simulink subsystem "MultibodySuspensionRearSSC"  (R2024b)
settings: Solver=VariableStepAuto  StartTime=0.0  StopTime=10.0  RelTol=1e-3
undefined symbols (not defined in the file): EnvGrvty, LAc, LAf, LAr, PlntVehDstCGFrntAxl, PlntVehDstCGRearAxl, PlntVehMass, PlntVehMultiBody, PlntVehMultiBodyGeom, RearRef, StrRodRL, UAc, UAf, UAr, Wheels, WhlAng, X, Y, Z
libraries: sm_lib x225, fl_lib x48, nesl_utility x32, sdl_lib x4
(part 1 of 9)
settings Model: ModifiedByFormat=The MathWorks, Inc.  Creator=The MathWorks, Inc.  LastModifiedBy=The MathWorks, Inc.
settings OptimizationCC: ReuseModelBlockBuffer=off
settings DebuggingCC: SubsystemReferenceDiagnosticForUnitTest=warning
settings RTWCC: GPUComputeCapability=3.5

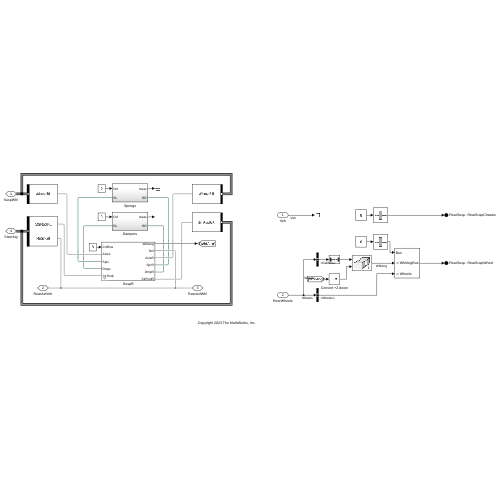
[thumbnail: Simulink's stored preview of the top-level diagram]
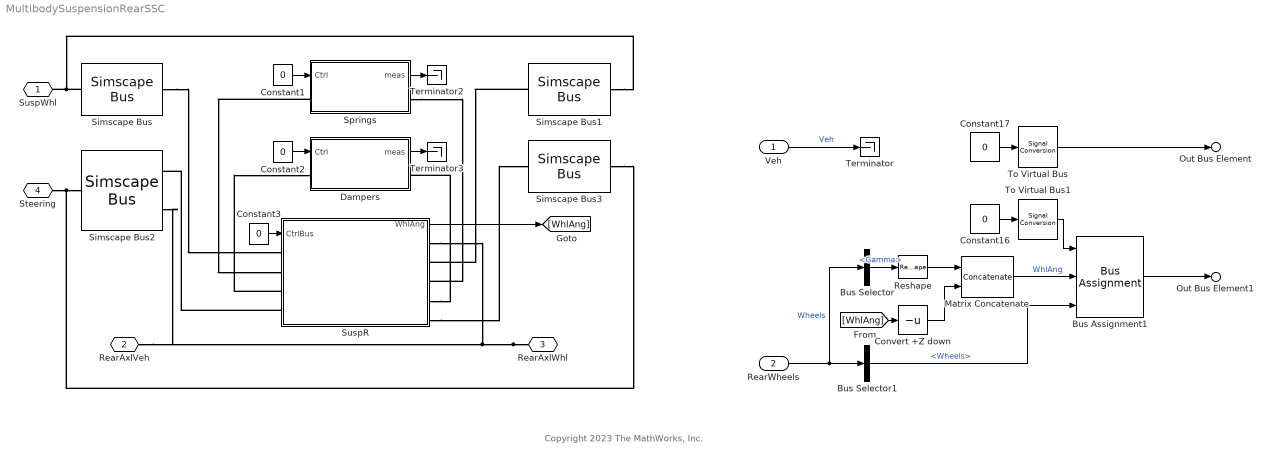
== system MultibodySuspensionRearSSC ==
  note: Copyright 2023 The MathWorks, Inc.
  Veh : Inport
  RearWheels : Inport  Port=2
  Bus Assignment1 : BusAssignment  AssignedSignals=WhlAng,Wheels
  Bus Selector : BusSelector  OutputSignals=Wheels.Gamma
  Bus Selector1 : BusSelector  OutputSignals=Wheels
  Constant1 : Constant  Value=0  SampleTime=-1
  Constant16 : Constant  Value=0  OutDataTypeStr=Bus: RearSuspWheelBUS  SampleTime=Inf
  Constant17 : Constant  Value=0  OutDataTypeStr=Bus: RearSuspChassisBUS  SampleTime=Inf
  Constant2 : Constant  Value=0  SampleTime=-1
  Constant3 : Constant  Value=0  SampleTime=-1
  Convert +Z down : UnaryMinus
  Dampers : Subsystem
  Matrix Concatenate : Concatenate  Mode=Multidimensional array
  Reshape : Reshape  OutputDimensionality=Row vector (2-D)
  Simscape Bus : SimscapeBus  HierarchyStrings=WheelRL
  Simscape Bus1 : SimscapeBus  HierarchyStrings=WheelRR
  Simscape Bus2 : SimscapeBus  HierarchyStrings=StrRodRL;RearRef
  Simscape Bus3 : SimscapeBus  HierarchyStrings=StrRodRR
  Springs : Subsystem
  SuspR : Subsystem  mask(Suspension and Steering){Susp=PlntVehMultiBody.Chassis.SuspR, Init=[0 0 0], InitTriggerDropdown=1}
      mask prompts: Susp "Suspension Parameters"; Init "Initial Values"; InitTriggerDropdown "Initialization Trigger Dropdown"
      mask help: Suspension and steering system for front or rear axle.
      mask init:
      | % curblk = gcb;
      | % Trigger Mask Initialization for 
      | % variant subsystems below this level
      | % sm_car_4post_lib_maskInitTrigger(curblk)
      settings: LibrarySourceBlock=sm_car_4post_lib/Suspension and Steering
      mask TypeOptions InitTriggerDropdown: 0 | 1
  Terminator : Terminator
  Terminator2 : Terminator
  Terminator3 : Terminator
  To Virtual Bus : SignalConversion  ConversionOutput=Virtual bus  OverrideOpt=off
  To Virtual Bus1 : SignalConversion  ConversionOutput=Virtual bus  OverrideOpt=off
  SuspWhl : PMIOPort  Side=Right
  RearAxlVeh : PMIOPort  Port=2  Side=Left
  RearAxlWhl : PMIOPort  Port=3  Side=Right
  Steering : PMIOPort  Port=4  Side=Left
  Out Bus Element : Outport  PortName=RearSusp  Element=RearSuspChassis
  Out Bus Element1 : Outport  PortName=RearSusp  Element=RearSuspWheel
  wires:
  Springs/1(meas) -> Terminator2/1
  Dampers/1(meas) -> Terminator3/1
  Constant1/1 -> Springs/1(Ctrl)
  Constant2/1 -> Dampers/1(Ctrl)
  Constant3/1 -> SuspR/1(CtrlBus)
  Bus Selector/1 -> Reshape/1  "<Gamma>"
  Reshape/1 -> Matrix Concatenate/1
  Convert +Z down/1 -> Matrix Concatenate/2
  SuspR/1(WhlAng) -> [WhlAng]
  [WhlAng] -> Convert +Z down/1
  Constant16/1 -> To Virtual Bus1/1
  To Virtual Bus/1 -> Out Bus Element/1
  Matrix Concatenate/1 -> Bus Assignment1/2  "WhlAng"
  Bus Assignment1/1 -> Out Bus Element1/1
  RearWheels/1 -> Bus Selector1/1, Bus Selector/1  "Wheels"
  Constant17/1 -> To Virtual Bus/1
  To Virtual Bus1/1 -> Bus Assignment1/1
  Bus Selector1/1 -> Bus Assignment1/3  "<Wheels>"
  Veh/1 -> Terminator/1  "Veh"
  connections:
  Steering/RConn1 -- Simscape Bus2/RConn1 -- Simscape Bus3/RConn1
  RearAxlWhl/RConn1 -- RearAxlVeh/RConn1 -- Simscape Bus2/LConn2 -- SuspR/RConn1
  Simscape Bus/RConn1 -- SuspWhl/RConn1 -- Simscape Bus1/RConn1
  SuspR/LConn4 -- Simscape Bus2/LConn1
  SuspR/RConn5 -- Simscape Bus3/LConn1
  Springs/LConn1 -- SuspR/LConn2
  Springs/RConn1 -- SuspR/RConn3
  SuspR/RConn4 -- Dampers/RConn1
  SuspR/LConn3 -- Dampers/LConn1
  Simscape Bus/LConn1 -- SuspR/LConn1
  Simscape Bus1/LConn1 -- SuspR/RConn2

== system MultibodySuspensionRearSSC/Dampers ==
  Ctrl : Inport
  Independent : Subsystem  VariantControl=Independent
  Terminator : Terminator
  RL : PMIOPort  Side=Left
  RR : PMIOPort  Port=2  Side=Right
  meas : Outport  VectorParamsAs1DForOutWhenUnconnected=off
  wires:
  Ctrl/1 -> Terminator/1
  Independent/1(meas) -> meas/1
  connections:
  Independent/RConn1 -- RR/RConn1
  Independent/LConn1 -- RL/RConn1

== system MultibodySuspensionRearSSC/Springs ==
  Ctrl : Inport
  Independent : Subsystem  VariantControl=Independent
  Terminator : Terminator
  RL : PMIOPort  Side=Left
  RR : PMIOPort  Port=2  Side=Right
  meas : Outport  VectorParamsAs1DForOutWhenUnconnected=off
  wires:
  Ctrl/1 -> Terminator/1
  Independent/1(meas) -> meas/1
  connections:
  Independent/RConn1 -- RR/RConn1
  Independent/LConn1 -- RL/RConn1

== system MultibodySuspensionRearSSC/SuspR ==
  CtrlBus : Inport
  Linkage : Subsystem  VariantControl=Linkage
  Terminator : Terminator
  AxleL : PMIOPort  Side=Left
  Ref : PMIOPort  Port=2  Side=Right
  AxleR : PMIOPort  Port=3  Side=Right
  SprL : PMIOPort  Port=4  Side=Left
  SprR : PMIOPort  Port=5  Side=Right
  DmpL : PMIOPort  Port=6  Side=Left
  DmpR : PMIOPort  Port=7  Side=Right
  StrRodL : PMIOPort  Port=8  Side=Left
  StrRodR : PMIOPort  Port=9  Side=Right
  WhlAng : Outport
  wires:
  Linkage/1(WhlAng) -> WhlAng/1
  CtrlBus/1 -> Terminator/1
  connections:
  Linkage/RConn5 -- StrRodR/RConn1
  StrRodL/RConn1 -- Linkage/LConn4
  Linkage/LConn1 -- AxleL/RConn1
  Linkage/RConn1 -- Ref/RConn1
  Linkage/RConn3 -- SprR/RConn1
  Linkage/RConn4 -- DmpR/RConn1
  Linkage/LConn2 -- SprL/RConn1
  Linkage/RConn2 -- AxleR/RConn1
  Linkage/LConn3 -- DmpL/RConn1

== system MultibodySuspensionRearSSC/Dampers/Independent ==
  Constant2 : Constant  Value=0  SampleTime=-1
  Constant3 : Constant  Value=0  SampleTime=-1
  Damper RL : Subsystem  mask(Damper){Damper=PlntVehMultiBody.Chassis.Damper.Rear}
      mask prompts: Damper "Damper Parameters"
      settings: LibrarySourceBlock=sm_car_4post_lib/Damper
  Damper RR : Subsystem  mask(Damper){Damper=PlntVehMultiBody.Chassis.Damper.Rear}
      mask prompts: Damper "Damper Parameters"
      settings: LibrarySourceBlock=sm_car_4post_lib/Damper
  MTRef RL : fl_lib/Mechanical/Translational Elements/Mechanical Translational Reference
  MTRef RR : fl_lib/Mechanical/Translational Elements/Mechanical Translational Reference
  RL : PMIOPort  Side=Left
  RR : PMIOPort  Port=2  Side=Right
  Out Bus Element2 : Outport  VectorParamsAs1DForOutWhenUnconnected=off  PortName=meas  Element=RL
  Out Bus Element3 : Outport  VectorParamsAs1DForOutWhenUnconnected=off  PortName=meas  Element=RR
  wires:
  Constant3/1 -> Damper RR/1(Ctrl)
  Constant2/1 -> Damper RL/1(Ctrl)
  Damper RR/1(meas) -> Out Bus Element3/1
  Damper RL/1(meas) -> Out Bus Element2/1
  connections:
  Damper RL/RConn1 -- MTRef RL/LConn1
  Damper RL/LConn1 -- RL/RConn1
  Damper RR/RConn1 -- MTRef RR/LConn1
  Damper RR/LConn1 -- RR/RConn1

== system MultibodySuspensionRearSSC/Springs/Independent ==
  Constant2 : Constant  Value=0  SampleTime=-1
  Constant3 : Constant  Value=0  SampleTime=-1
  MTRef RL : fl_lib/Mechanical/Translational Elements/Mechanical Translational Reference
  MTRef RR : fl_lib/Mechanical/Translational Elements/Mechanical Translational Reference
  Spring RL : Subsystem  mask(Spring){Spring=PlntVehMultiBody.Chassis.Spring.Rear}
      mask prompts: Spring "Spring Parameters"
      settings: LibrarySourceBlock=sm_car_4post_lib/Spring
  Spring RR : Subsystem  mask(Spring){Spring=PlntVehMultiBody.Chassis.Spring.Rear}
      mask prompts: Spring "Spring Parameters"
      settings: LibrarySourceBlock=sm_car_4post_lib/Spring
  RL : PMIOPort  Side=Left
  RR : PMIOPort  Port=2  Side=Right
  Out Bus Element2 : Outport  VectorParamsAs1DForOutWhenUnconnected=off  PortName=meas  Element=RL
  Out Bus Element3 : Outport  VectorParamsAs1DForOutWhenUnconnected=off  PortName=meas  Element=RR
  wires:
  Constant3/1 -> Spring RR/1(Ctrl)
  Constant2/1 -> Spring RL/1(Ctrl)
  Spring RR/1(meas) -> Out Bus Element3/1
  Spring RL/1(meas) -> Out Bus Element2/1
  connections:
  Spring RL/RConn1 -- MTRef RL/LConn1
  Spring RL/LConn1 -- RL/RConn1
  Spring RR/RConn1 -- MTRef RR/LConn1
  Spring RR/LConn1 -- RR/RConn1

== system MultibodySuspensionRearSSC/SuspR/Linkage ==
  Anti Roll Bar : Subsystem  Variant=on  VariantControlMode=label  LabelModeActiveChoice=Simple  mask{AntiRollBar=Susp.AntiRollBar, VariantLabel=Susp.AntiRollBar.class.Value, InitTriggerDropdown=1}
      mask prompts: AntiRollBar "Anti-Roll Bar"; VariantLabel "Variant Label"; InitTriggerDropdown "Initialization Trigger Dropdown"
      settings: AttributesFormatString=%<LabelModeActiveChoice>
      mask TypeOptions InitTriggerDropdown: 0 | 1
  Linkage L : Subsystem  Variant=on  VariantControlMode=label  VariantControl=Variant1  LabelModeActiveChoice=DoubleWishbone  mask(Suspension){popup_leftRight=Left, Linkage=Susp.Linkage, Init=[0 0 0], VariantLabel=Susp.Linkage.class.Value, InitTriggerDropdown=1}
      mask prompts: popup_leftRight "Left/Right"; Linkage "Linkage Parameters"; Init "Initial Values"; VariantLabel "Variant Label"; InitTriggerDropdown "Initialization Trigger Dropdown"
      mask help: Suspension with multiple variants. Variants are configured by parameter Variant Label. Parameter values are contained within Linkage Parameters.
      mask init:
      | % curblk = gcb;
      | 
      | % Set variant for this block 
      | % set_param(curblk,'LabelModeActiveChoice',VariantLabel);
      | 
      | % Trigger Mask Initialization for 
      | % variant subsystems below this level
      | % sm_car_4post_lib_maskInitTrigger(curblk)
      | 
      | % Set Left/Right fields
      | 
      | % sm_car_4post_lib_setLeftRight(curblk,'variant');
      settings: AttributesFormatString=%<ActiveVariant>  LibrarySourceBlock=sm_car_4post_lib/Suspension and Steering/Linkage/Linkage L
      mask TypeOptions popup_leftRight: Left | Right
      mask TypeOptions InitTriggerDropdown: 0 | 1
  Linkage R : Subsystem  Variant=on  VariantControlMode=label  VariantControl=Variant1  LabelModeActiveChoice=DoubleWishbone  mask(Suspension){popup_leftRight=Right, Linkage=Susp.Linkage, Init=[0 0 0], VariantLabel=Susp.Linkage.class.Value, InitTriggerDropdown=1}
      mask prompts: popup_leftRight "Left/Right"; Linkage "Linkage Parameters"; Init "Initial Values"; VariantLabel "Variant Label"; InitTriggerDropdown "Initialization Trigger Dropdown"
      mask help: Suspension with multiple variants. Variants are configured by parameter Variant Label. Parameter values are contained within Linkage Parameters.
      mask init:
      | % curblk = gcb;
      | 
      | % % Set variant for this block 
      | % set_param(curblk,'LabelModeActiveChoice',VariantLabel);
      | 
      | % Trigger Mask Initialization for 
      | % variant subsystems below this level
      | % sm_car_4post_lib_maskInitTrigger(curblk)
      | 
      | % Set Left/Right fields
      | 
      | % sm_car_4post_lib_setLeftRight(curblk,'variant');
      settings: AttributesFormatString=%<ActiveVariant>  LibrarySourceBlock=sm_car_4post_lib/Suspension and Steering/Linkage/Linkage R
      mask TypeOptions popup_leftRight: Left | Right
      mask TypeOptions InitTriggerDropdown: 0 | 1
  Matrix Concatenate : Concatenate  Mode=Multidimensional array  ConcatenateDimension=2
  AxleL : PMIOPort  Side=Left
  Ref : PMIOPort  Port=2  Side=Right
  AxleR : PMIOPort  Port=3  Side=Right
  SprL : PMIOPort  Port=4  Side=Left
  SprR : PMIOPort  Port=5  Side=Right
  DmpL : PMIOPort  Port=6  Side=Left
  DmpR : PMIOPort  Port=7  Side=Right
  StrRodL : PMIOPort  Port=8  Side=Left
  StrRodR : PMIOPort  Port=9  Side=Right
  WhlAng : Outport
  wires:
  Matrix Concatenate/1 -> WhlAng/1
  Linkage R/1(WhlAng) -> Matrix Concatenate/2
  Linkage L/1(WhlAng) -> Matrix Concatenate/1
  connections:
  Anti Roll Bar/LConn3 -- Linkage R/LConn4
  Anti Roll Bar/LConn1 -- Linkage L/LConn4
  Linkage R/LConn2 -- SprR/RConn1
  Linkage R/LConn3 -- DmpR/RConn1
  Linkage R/RConn1 -- StrRodR/RConn1
  Ref/RConn1 -- Anti Roll Bar/LConn2 -- Linkage L/RConn2 -- Linkage R/RConn2
  Linkage L/LConn1 -- AxleL/RConn1
  Linkage R/LConn1 -- AxleR/RConn1
  Linkage L/LConn2 -- SprL/RConn1
  Linkage L/LConn3 -- DmpL/RConn1
  Linkage L/RConn1 -- StrRodL/RConn1

== system MultibodySuspensionRearSSC/Dampers/Independent/Damper RL ==
  Ctrl : Inport
  Damper : Subsystem  Variant=on  VariantControlMode=label  VariantControl=Linear  LabelModeActiveChoice=Linear
  R : PMIOPort  Side=Left
  C : PMIOPort  Port=2  Side=Right
  meas : Outport  VectorParamsAs1DForOutWhenUnconnected=off
  wires:
  Damper/1(meas) -> meas/1
  Ctrl/1 -> Damper/1(Ctrl)
  connections:
  Damper/LConn1 -- R/RConn1
  Damper/RConn1 -- C/RConn1

== system MultibodySuspensionRearSSC/Dampers/Independent/Damper RR ==
  Ctrl : Inport
  Damper : Subsystem  Variant=on  VariantControlMode=label  VariantControl=Linear  LabelModeActiveChoice=Linear
  R : PMIOPort  Side=Left
  C : PMIOPort  Port=2  Side=Right
  meas : Outport  VectorParamsAs1DForOutWhenUnconnected=off
  wires:
  Damper/1(meas) -> meas/1
  Ctrl/1 -> Damper/1(Ctrl)
  connections:
  Damper/LConn1 -- R/RConn1
  Damper/RConn1 -- C/RConn1

== system MultibodySuspensionRearSSC/Springs/Independent/Spring RL ==
  Ctrl : Inport
  Spring : Subsystem  Variant=on  VariantControlMode=label  VariantControl=Linear  LabelModeActiveChoice=Linear
  R : PMIOPort  Side=Left
  C : PMIOPort  Port=2  Side=Right
  meas : Outport  VectorParamsAs1DForOutWhenUnconnected=off
  wires:
  Ctrl/1 -> Spring/1(Ctrl)
  Spring/1(meas) -> meas/1
  connections:
  Spring/RConn1 -- C/RConn1
  Spring/LConn1 -- R/RConn1

== system MultibodySuspensionRearSSC/Springs/Independent/Spring RR ==
  Ctrl : Inport
  Spring : Subsystem  Variant=on  VariantControlMode=label  VariantControl=Linear  LabelModeActiveChoice=Linear
  R : PMIOPort  Side=Left
  C : PMIOPort  Port=2  Side=Right
  meas : Outport  VectorParamsAs1DForOutWhenUnconnected=off
  wires:
  Ctrl/1 -> Spring/1(Ctrl)
  Spring/1(meas) -> meas/1
  connections:
  Spring/RConn1 -- C/RConn1
  Spring/LConn1 -- R/RConn1

== system MultibodySuspensionRearSSC/SuspR/Linkage/Anti Roll Bar ==
  " None" : Subsystem  VariantControl=None  mask(Anti-Roll Bar Placeholder){}
      mask help: Empty subsystem, used as a variant that omits an anti-roll bar.
  Simple : Subsystem  VariantControl=Simple  mask(Anti-Roll Bar, Simple){k=AntiRollBar.k.Value}
      mask prompts: k "Stiffness"
      mask help: Models an anti-roll bar by applying un-opposed forces to suspension arms. Conceptual use only.
  LAoL : PMIOPort  Side=Left
  Ref : PMIOPort  Port=2  Side=Left
  LAoR : PMIOPort  Port=3  Side=Left

== system MultibodySuspensionRearSSC/SuspR/Linkage/Linkage L ==
  DoubleWishbone : Subsystem  VariantControl=DoubleWishbone  mask(Double-Wishbone Suspension){popup_leftRight=Left, hp_in_f_ua=Linkage.UpperWishbone.sInboardF.Value, hp_in_r_ua=Linkage.UpperWishbone.sInboardR.Value, hp_out_ua=Linkage.UpperWishbone.sOutboard.Value, hp_in_f_la=Linkage.LowerWishbone.sInboardF.Value, hp_in_r_la=Linkage.LowerWishbone.sInboardR.Value, hp_out_la=Linkage.LowerWishbone.sOutboard.Value, hp_upr_cg=Linkage.Upright.sCG.Value, hp_upr_wc=Linkage.Upright.sWheelCentre.Value, hp_in_rod=Linkage.TrackRod.sInboard.Value, hp_upr_rod=Linkage.TrackRod.sOutboard.Value, hp_spr_top=Linkage.Shock.sTop.Value, hp_spr_bot=Linkage.Shock.sBottom.Value, clr_hp=PlntVehMultiBodyGeom.hp.clr, opc_hp=PlntVehMultiBodyGeom.hp.opc, size_hp=0.025, ua_mass=Linkage.UpperWishbone.m.Value, clr_ua=PlntVehMultiBodyGeom.yellow, opc_ua=PlntVehMultiBodyGeom.part.opc, radius_ua=0.02, la_mass=Linkage.LowerWishbone.m.Value, clr_la=PlntVehMultiBodyGeom.yellow, opc_la=PlntVehMultiBodyGeom.part.opc, radius_la=0.02, shock_pist_mass=Linkage.Shock.mPiston.Value, shock_cyl_mass=Linkage.Shock.mCylinder.Value, up_lim_bumpstop=Linkage.Endstop.xMax.Value, low_lim_bumpstop=Linkage.Endstop.xMin.Value, clr_conn_shock=PlntVehMultiBodyGeom.hp.clr, opc_conn_shock=PlntVehMultiBodyGeom.hp.opc, size_conn_shock=0.025, clr_shock_cyl=PlntVehMultiBodyGeom.blue, opc_shock_cyl=1.0, radius_shock_cyl=0.05, clr_shock_piston=PlntVehMultiBodyGeom.gray, opc_shock_piston=1.0, clr_shock_bumpstop=PlntVehMultiBodyGeom.yellowpale, opc_shock_bumpstop=1.0, deadvol_len_shock_cyl=PlntVehMultiBodyGeom.shock.dead_length, piston_len_shock=PlntVehMultiBodyGeom.shock.piston, cyl_cap_len_shock=PlntVehMultiBodyGeom.shock.cap, bumpstop_len_shock=PlntVehMultiBodyGeom.shock.bumpstop_len, upr_mass=Linkage.Upright.m.Value, atoe=Linkage.Upright.aToe.Value, acamber=Linkage.Upright.aCamber.Value, clr_conn_upr=PlntVehMultiBodyGeom.hp.clr, opc_conn_upr=PlntVehMultiBodyGeom.hp.opc, size_conn_upr=PlntVehMultiBodyGeom.hp.rad, clr_upr=PlntVehMultiBodyGeom.green, opc_upr=PlntVehMultiBodyGeom.part.opc, radius_upr=0.02, clr_stub_axle=PlntVehMultiBodyGeom.black, opc_stub_axle=PlntVehMultiBodyGeom.part.opc, radius_stub_axle=0.02, rod_mass=Linkage.TrackRod.m.Value, clr_conn_rod=PlntVehMultiBodyGeom.hp.clr, opc_conn_rod=PlntVehMultiBodyGeom.hp.opc, size_conn_rod=PlntVehMultiBodyGeom.hp.rad, clr_rod=PlntVehMultiBodyGeom.purple, opc_rod=PlntVehMultiBodyGeom.part.opc, radius_rod=0.02, whl_init_spd_lr=[0 0 0], whlind=1}
      mask prompts: popup_leftRight "Left/Right"; hp_in_f_ua "Upper Arm Front [xyz] (m)"; hp_in_r_ua "Upper Arm Rear [xyz] (m)"; hp_out_ua "Upper Arm Outboard [xyz] (m)"; hp_in_f_la "Lower Arm Front [xyz] (m)"; hp_in_r_la "Lower Arm Rear [xyz] (m)"; hp_out_la "Lower Arm Outboard [xyz] (m)"; hp_upr_cg "Upright CG [xyz] (m)"; hp_upr_wc "Wheel Center [xyz] (m)"; hp_in_rod "Track Rod Inboard [xyz] (m)"; hp_upr_rod "Track Rod Outboard [xyz] (m)"; hp_spr_top "Spring Top [xyz] (m)"; hp_spr_bot "Spring Bottom [xyz] (m)"; ua_mass "Mass (kg)"; clr_ua "Color [RGB]"; opc_ua "Opacity (0-1)"; radius_ua "Radius (m)"; la_mass "Mass (kg)"; clr_la "Color [RGB]"; opc_la "Opacity (0-1)"; radius_la "Radius (m)"; shock_pist_mass "Piston Mass (kg)"; shock_cyl_mass "Cylinder Mass (kg)"; up_lim_bumpstop "Upper Limit (m)"; low_lim_bumpstop "Lower Limit (m)"; deadvol_len_shock_cyl "Dead Volume Height (m)"; piston_len_shock "Piston Length (m)"; cyl_cap_len_shock "Cylinder Cap Length (m)"; bumpstop_len_shock "Bumpstop Length (m)"; upr_mass "Mass (kg)"; atoe "Toe Angle (deg)"; acamber "Camber Angle (deg)"; rod_mass "Mass (kg)"; whl_init_spd_lr "Initial Wheel Speed (rad/s)"; whlind "Wheel Index"
      mask help: This models a double-wishbone suspension for steered and non-steered configurations. The non-steered configuration maintains its orientation via the track rods that connect to fixed points on the subframe.
      mask init:
      | % sm_car_4post_lib_setLeftRight(gcb,'none');
      | 
      | if(popup_leftRight == 1)
      |     rhs_susp = 1;
      |     whlind = 1;
      | elseif(popup_leftRight == 2)
      |     rhs_susp = -1;
      |     whlind = 2;
      | end
      mask TypeOptions popup_leftRight: Left | Right
      mask TypeOptions hp_in_f_ua: Upper Arm/hp_in_f | Hardpoints/hp_in_f_ua
      mask TypeOptions hp_in_r_ua: Upper Arm/hp_in_r | Hardpoints/hp_in_r_ua
      mask TypeOptions hp_out_ua: Upper Arm/hp_out | Upright/hp_ua_out
      mask TypeOptions hp_in_f_la: Lower Arm/hp_in_f | Hardpoints/hp_in_f_la
      mask TypeOptions hp_in_r_la: Lower Arm/hp_in_r | Hardpoints/hp_in_r_la
      mask TypeOptions hp_out_la: Lower Arm/hp_out | Upright/hp_la_out
      mask TypeOptions hp_upr_cg: Upright/hp_upr_cg
      mask TypeOptions hp_upr_wc: Upright/hp_upr_wc
      mask TypeOptions hp_in_rod: Track Rod/hp_in
      mask TypeOptions hp_upr_rod: Track Rod/hp_out | Upright/hp_upr_rod
      mask TypeOptions hp_spr_top: Hardpoints/hp_spr_top | Shock/hp_spr_top
      mask TypeOptions hp_spr_bot: Lower Arm/hp_spr | Shock/hp_spr_bot
      mask TypeOptions clr_hp: Hardpoints/clr_hp
      mask TypeOptions opc_hp: Hardpoints/opc_hp
      mask TypeOptions size_hp: Hardpoints/size_hp
      mask TypeOptions ua_mass: Upper Arm/ua_mass
      mask TypeOptions clr_ua: Upper Arm/clr_ua
      mask TypeOptions opc_ua: Upper Arm/opc_ua
      mask TypeOptions radius_ua: Upper Arm/radius_ua
      mask TypeOptions la_mass: Lower Arm/la_mass
      mask TypeOptions clr_la: Lower Arm/clr_la
      mask TypeOptions opc_la: Lower Arm/opc_la
      mask TypeOptions radius_la: Lower Arm/radius_la
      mask TypeOptions shock_pist_mass: Shock/shock_pist_mass
      mask TypeOptions shock_cyl_mass: Shock/shock_cyl_mass
      mask TypeOptions up_lim_bumpstop: Shock/up_lim_bumpstop
      mask TypeOptions low_lim_bumpstop: Shock/low_lim_bumpstop
      mask TypeOptions clr_conn_shock: Shock/clr_conn_shock
      mask TypeOptions opc_conn_shock: Shock/opc_conn_shock
      mask TypeOptions size_conn_shock: Shock/size_conn_shock
      mask TypeOptions clr_shock_cyl: Shock/clr_shock_cyl
      mask TypeOptions opc_shock_cyl: Shock/opc_shock_cyl
      mask TypeOptions radius_shock_cyl: Shock/radius_shock_cyl
      mask TypeOptions clr_shock_piston: Shock/clr_shock_piston
      mask TypeOptions opc_shock_piston: Shock/opc_shock_piston
      mask TypeOptions clr_shock_bumpstop: Shock/clr_shock_bumpstop
      mask TypeOptions opc_shock_bumpstop: Shock/opc_shock_bumpstop
      mask TypeOptions deadvol_len_shock_cyl: Shock/deadvol_len_shock_cyl
      mask TypeOptions piston_len_shock: Shock/piston_len_shock
      mask TypeOptions cyl_cap_len_shock: Shock/cyl_cap_len_shock
      mask TypeOptions bumpstop_len_shock: Shock/bumpstop_len_shock
      mask TypeOptions upr_mass: Upright/upr_mass
      mask TypeOptions atoe: Upright/atoe
      mask TypeOptions acamber: Upright/acamber
      mask TypeOptions clr_conn_upr: Upright/clr_conn_upr
      mask TypeOptions opc_conn_upr: Upright/opc_conn_upr
      mask TypeOptions size_conn_upr: Upright/size_conn_upr
      mask TypeOptions clr_upr: Upright/clr_upr
      mask TypeOptions opc_upr: Upright/opc_upr
      mask TypeOptions radius_upr: Upright/radius_upr
      mask TypeOptions clr_stub_axle: Upright/clr_stub_axle
      mask TypeOptions opc_stub_axle: Upright/opc_stub_axle
      mask TypeOptions radius_stub_axle: Upright/radius_stub_axle
      mask TypeOptions rod_mass: Track Rod/rod_mass
      mask TypeOptions clr_conn_rod: Track Rod/clr_conn_rod
      mask TypeOptions opc_conn_rod: Track Rod/opc_conn_rod
      mask TypeOptions size_conn_rod: Track Rod/size_conn_rod
      mask TypeOptions clr_rod: Track Rod/clr_rod
      mask TypeOptions opc_rod: Track Rod/opc_rod
      mask TypeOptions radius_rod: Track Rod/radius_rod
      mask DialogControl cont_hp Prompt: Hardpoints
      mask DialogControl cont_vis_hp Prompt: Visualization
      mask DialogControl text_clr_hp Prompt: Color [RGB]
      mask DialogControl text_opc_hp Prompt: Opac. (0-1)
      mask DialogControl text_size_hp Prompt: Size (m)
      mask DialogControl text_hp Prompt: Hardpoints
      mask DialogControl cont_ua Prompt: UA
      mask DialogControl cont_vis_ua Prompt: Visualization
      mask DialogControl cont_la Prompt: LA
      mask DialogControl cont_vis_la Prompt: Visualization
      mask DialogControl cont_shock Prompt: Shock
      mask DialogControl cont_parts Prompt: Parts
      mask DialogControl cont_bumpstop Prompt: Bumpstop
      mask DialogControl cont_vis_shock Prompt: Visualization
      mask DialogControl text_clr_shock Prompt: Color  [RGB]
      mask DialogControl text_opc_shock Prompt: Opac. (0-1)
      mask DialogControl text_size_shock Prompt: Size (m)
      mask DialogControl text_conn_shock Prompt: Connections
      mask DialogControl text_shock_shock Prompt: Cylinder
      mask DialogControl text_shock_piston Prompt: Piston
      mask DialogControl text_piston_radius Prompt: <cylinder radius>
      mask DialogControl text_shock_bumpstop Prompt: Bumpstop
      mask DialogControl text_bumpstop_radius Prompt: <cylinder radius>
      mask DialogControl cont_upright Prompt: Upright
      mask DialogControl grp_upright Prompt: Upright
      mask DialogControl cont_vis_upr Prompt: Visualization
      mask DialogControl text_clr_upr Prompt: Color [RGB]
      mask DialogControl text_opc_upr Prompt: Opac. (0-1)
      mask DialogControl text_size_upr Prompt: Size (m)
      mask DialogControl text_conn_upr Prompt: Connections
      mask DialogControl text_upright Prompt: Upright
      mask DialogControl text_stub_axle Prompt: Stub Axle
      mask DialogControl cont_steer Prompt: Steer
      mask DialogControl grp_rod Prompt: Rod
      mask DialogControl cont_vis_rod Prompt: Visualization
      mask DialogControl text_clr_rod Prompt: Color [RGB]
      mask DialogControl text_opc_rod Prompt: Opac. (0-1)
      mask DialogControl text_size_rod Prompt: Size (m)
      mask DialogControl text_conn_rod Prompt: Connections
      mask DialogControl text_rod_rod Prompt: Rod
      mask DialogControl cont_init Prompt: Initial
  Rack : PMIOPort  Side=Right
  Ref : PMIOPort  Port=2  Side=Right
  Axle : PMIOPort  Port=3  Side=Left
  S : PMIOPort  Port=4  Side=Left
  D : PMIOPort  Port=5  Side=Left
  LAo : PMIOPort  Port=6  Side=Left
  WhlAng : Outport

== system MultibodySuspensionRearSSC/SuspR/Linkage/Linkage R ==
  DoubleWishbone : Subsystem  VariantControl=DoubleWishbone  mask(Double-Wishbone Suspension){popup_leftRight=Right, hp_in_f_ua=Linkage.UpperWishbone.sInboardF.Value, hp_in_r_ua=Linkage.UpperWishbone.sInboardR.Value, hp_out_ua=Linkage.UpperWishbone.sOutboard.Value, hp_in_f_la=Linkage.LowerWishbone.sInboardF.Value, hp_in_r_la=Linkage.LowerWishbone.sInboardR.Value, hp_out_la=Linkage.LowerWishbone.sOutboard.Value, hp_upr_cg=Linkage.Upright.sCG.Value, hp_upr_wc=Linkage.Upright.sWheelCentre.Value, hp_in_rod=Linkage.TrackRod.sInboard.Value, hp_upr_rod=Linkage.TrackRod.sOutboard.Value, hp_spr_top=Linkage.Shock.sTop.Value, hp_spr_bot=Linkage.Shock.sBottom.Value, clr_hp=PlntVehMultiBodyGeom.hp.clr, opc_hp=PlntVehMultiBodyGeom.hp.opc, size_hp=0.025, ua_mass=Linkage.UpperWishbone.m.Value, clr_ua=PlntVehMultiBodyGeom.yellow, opc_ua=PlntVehMultiBodyGeom.part.opc, radius_ua=0.02, la_mass=Linkage.LowerWishbone.m.Value, clr_la=PlntVehMultiBodyGeom.yellow, opc_la=PlntVehMultiBodyGeom.part.opc, radius_la=0.02, shock_pist_mass=Linkage.Shock.mPiston.Value, shock_cyl_mass=Linkage.Shock.mCylinder.Value, up_lim_bumpstop=Linkage.Endstop.xMax.Value, low_lim_bumpstop=Linkage.Endstop.xMin.Value, clr_conn_shock=PlntVehMultiBodyGeom.hp.clr, opc_conn_shock=PlntVehMultiBodyGeom.hp.opc, size_conn_shock=0.025, clr_shock_cyl=PlntVehMultiBodyGeom.blue, opc_shock_cyl=1.0, radius_shock_cyl=0.05, clr_shock_piston=PlntVehMultiBodyGeom.gray, opc_shock_piston=1.0, clr_shock_bumpstop=PlntVehMultiBodyGeom.yellowpale, opc_shock_bumpstop=1.0, deadvol_len_shock_cyl=PlntVehMultiBodyGeom.shock.dead_length, piston_len_shock=PlntVehMultiBodyGeom.shock.piston, cyl_cap_len_shock=PlntVehMultiBodyGeom.shock.cap, bumpstop_len_shock=PlntVehMultiBodyGeom.shock.bumpstop_len, upr_mass=Linkage.Upright.m.Value, atoe=Linkage.Upright.aToe.Value, acamber=Linkage.Upright.aCamber.Value, clr_conn_upr=PlntVehMultiBodyGeom.hp.clr, opc_conn_upr=PlntVehMultiBodyGeom.hp.opc, size_conn_upr=PlntVehMultiBodyGeom.hp.rad, clr_upr=PlntVehMultiBodyGeom.green, opc_upr=PlntVehMultiBodyGeom.part.opc, radius_upr=0.02, clr_stub_axle=PlntVehMultiBodyGeom.black, opc_stub_axle=PlntVehMultiBodyGeom.part.opc, radius_stub_axle=0.02, rod_mass=Linkage.TrackRod.m.Value, clr_conn_rod=PlntVehMultiBodyGeom.hp.clr, opc_conn_rod=PlntVehMultiBodyGeom.hp.opc, size_conn_rod=PlntVehMultiBodyGeom.hp.rad, clr_rod=PlntVehMultiBodyGeom.purple, opc_rod=PlntVehMultiBodyGeom.part.opc, radius_rod=0.02, whl_init_spd_lr=[0 0 0], whlind=1}
      mask prompts: popup_leftRight "Left/Right"; hp_in_f_ua "Upper Arm Front [xyz] (m)"; hp_in_r_ua "Upper Arm Rear [xyz] (m)"; hp_out_ua "Upper Arm Outboard [xyz] (m)"; hp_in_f_la "Lower Arm Front [xyz] (m)"; hp_in_r_la "Lower Arm Rear [xyz] (m)"; hp_out_la "Lower Arm Outboard [xyz] (m)"; hp_upr_cg "Upright CG [xyz] (m)"; hp_upr_wc "Wheel Center [xyz] (m)"; hp_in_rod "Track Rod Inboard [xyz] (m)"; hp_upr_rod "Track Rod Outboard [xyz] (m)"; hp_spr_top "Spring Top [xyz] (m)"; hp_spr_bot "Spring Bottom [xyz] (m)"; ua_mass "Mass (kg)"; clr_ua "Color [RGB]"; opc_ua "Opacity (0-1)"; radius_ua "Radius (m)"; la_mass "Mass (kg)"; clr_la "Color [RGB]"; opc_la "Opacity (0-1)"; radius_la "Radius (m)"; shock_pist_mass "Piston Mass (kg)"; shock_cyl_mass "Cylinder Mass (kg)"; up_lim_bumpstop "Upper Limit (m)"; low_lim_bumpstop "Lower Limit (m)"; deadvol_len_shock_cyl "Dead Volume Height (m)"; piston_len_shock "Piston Length (m)"; cyl_cap_len_shock "Cylinder Cap Length (m)"; bumpstop_len_shock "Bumpstop Length (m)"; upr_mass "Mass (kg)"; atoe "Toe Angle (deg)"; acamber "Camber Angle (deg)"; rod_mass "Mass (kg)"; whl_init_spd_lr "Initial Wheel Speed (rad/s)"; whlind "Wheel Index"
      mask help: This models a double-wishbone suspension for steered and non-steered configurations. The non-steered configuration maintains its orientation via the track rods that connect to fixed points on the subframe.
      mask init:
      | % sm_car_4post_lib_setLeftRight(gcb,'none');
      | 
      | if(popup_leftRight == 1)
      |     rhs_susp = 1;
      |     whlind = 1;
      | elseif(popup_leftRight == 2)
      |     rhs_susp = -1;
      |     whlind = 2;
      | end
      mask TypeOptions popup_leftRight: Left | Right
      mask TypeOptions hp_in_f_ua: Upper Arm/hp_in_f | Hardpoints/hp_in_f_ua
      mask TypeOptions hp_in_r_ua: Upper Arm/hp_in_r | Hardpoints/hp_in_r_ua
      mask TypeOptions hp_out_ua: Upper Arm/hp_out | Upright/hp_ua_out
      mask TypeOptions hp_in_f_la: Lower Arm/hp_in_f | Hardpoints/hp_in_f_la
      mask TypeOptions hp_in_r_la: Lower Arm/hp_in_r | Hardpoints/hp_in_r_la
      mask TypeOptions hp_out_la: Lower Arm/hp_out | Upright/hp_la_out
      mask TypeOptions hp_upr_cg: Upright/hp_upr_cg
      mask TypeOptions hp_upr_wc: Upright/hp_upr_wc
      mask TypeOptions hp_in_rod: Track Rod/hp_in
      mask TypeOptions hp_upr_rod: Track Rod/hp_out | Upright/hp_upr_rod
      mask TypeOptions hp_spr_top: Hardpoints/hp_spr_top | Shock/hp_spr_top
      mask TypeOptions hp_spr_bot: Lower Arm/hp_spr | Shock/hp_spr_bot
      mask TypeOptions clr_hp: Hardpoints/clr_hp
      mask TypeOptions opc_hp: Hardpoints/opc_hp
      mask TypeOptions size_hp: Hardpoints/size_hp
      mask TypeOptions ua_mass: Upper Arm/ua_mass
      mask TypeOptions clr_ua: Upper Arm/clr_ua
      mask TypeOptions opc_ua: Upper Arm/opc_ua
      mask TypeOptions radius_ua: Upper Arm/radius_ua
      mask TypeOptions la_mass: Lower Arm/la_mass
      mask TypeOptions clr_la: Lower Arm/clr_la
      mask TypeOptions opc_la: Lower Arm/opc_la
      mask TypeOptions radius_la: Lower Arm/radius_la
      mask TypeOptions shock_pist_mass: Shock/shock_pist_mass
      mask TypeOptions shock_cyl_mass: Shock/shock_cyl_mass
      mask TypeOptions up_lim_bumpstop: Shock/up_lim_bumpstop
      mask TypeOptions low_lim_bumpstop: Shock/low_lim_bumpstop
      mask TypeOptions clr_conn_shock: Shock/clr_conn_shock
      mask TypeOptions opc_conn_shock: Shock/opc_conn_shock
      mask TypeOptions size_conn_shock: Shock/size_conn_shock
      mask TypeOptions clr_shock_cyl: Shock/clr_shock_cyl
      mask TypeOptions opc_shock_cyl: Shock/opc_shock_cyl
      mask TypeOptions radius_shock_cyl: Shock/radius_shock_cyl
      mask TypeOptions clr_shock_piston: Shock/clr_shock_piston
      mask TypeOptions opc_shock_piston: Shock/opc_shock_piston
      mask TypeOptions clr_shock_bumpstop: Shock/clr_shock_bumpstop
      mask TypeOptions opc_shock_bumpstop: Shock/opc_shock_bumpstop
      mask TypeOptions deadvol_len_shock_cyl: Shock/deadvol_len_shock_cyl
      mask TypeOptions piston_len_shock: Shock/piston_len_shock
      mask TypeOptions cyl_cap_len_shock: Shock/cyl_cap_len_shock
      mask TypeOptions bumpstop_len_shock: Shock/bumpstop_len_shock
      mask TypeOptions upr_mass: Upright/upr_mass
      mask TypeOptions atoe: Upright/atoe
      mask TypeOptions acamber: Upright/acamber
      mask TypeOptions clr_conn_upr: Upright/clr_conn_upr
      mask TypeOptions opc_conn_upr: Upright/opc_conn_upr
      mask TypeOptions size_conn_upr: Upright/size_conn_upr
      mask TypeOptions clr_upr: Upright/clr_upr
      mask TypeOptions opc_upr: Upright/opc_upr
      mask TypeOptions radius_upr: Upright/radius_upr
      mask TypeOptions clr_stub_axle: Upright/clr_stub_axle
      mask TypeOptions opc_stub_axle: Upright/opc_stub_axle
      mask TypeOptions radius_stub_axle: Upright/radius_stub_axle
      mask TypeOptions rod_mass: Track Rod/rod_mass
      mask TypeOptions clr_conn_rod: Track Rod/clr_conn_rod
      mask TypeOptions opc_conn_rod: Track Rod/opc_conn_rod
      mask TypeOptions size_conn_rod: Track Rod/size_conn_rod
      mask TypeOptions clr_rod: Track Rod/clr_rod
      mask TypeOptions opc_rod: Track Rod/opc_rod
      mask TypeOptions radius_rod: Track Rod/radius_rod
      mask DialogControl cont_hp Prompt: Hardpoints
      mask DialogControl cont_vis_hp Prompt: Visualization
      mask DialogControl text_clr_hp Prompt: Color [RGB]
      mask DialogControl text_opc_hp Prompt: Opac. (0-1)
      mask DialogControl text_size_hp Prompt: Size (m)
      mask DialogControl text_hp Prompt: Hardpoints
      mask DialogControl cont_ua Prompt: UA
      mask DialogControl cont_vis_ua Prompt: Visualization
      mask DialogControl cont_la Prompt: LA
      mask DialogControl cont_vis_la Prompt: Visualization
      mask DialogControl cont_shock Prompt: Shock
      mask DialogControl cont_parts Prompt: Parts
      mask DialogControl cont_bumpstop Prompt: Bumpstop
      mask DialogControl cont_vis_shock Prompt: Visualization
      mask DialogControl text_clr_shock Prompt: Color  [RGB]
      mask DialogControl text_opc_shock Prompt: Opac. (0-1)
      mask DialogControl text_size_shock Prompt: Size (m)
      mask DialogControl text_conn_shock Prompt: Connections
      mask DialogControl text_shock_shock Prompt: Cylinder
      mask DialogControl text_shock_piston Prompt: Piston
      mask DialogControl text_piston_radius Prompt: <cylinder radius>
      mask DialogControl text_shock_bumpstop Prompt: Bumpstop
      mask DialogControl text_bumpstop_radius Prompt: <cylinder radius>
      mask DialogControl cont_upright Prompt: Upright
      mask DialogControl grp_upright Prompt: Upright
      mask DialogControl cont_vis_upr Prompt: Visualization
      mask DialogControl text_clr_upr Prompt: Color [RGB]
      mask DialogControl text_opc_upr Prompt: Opac. (0-1)
      mask DialogControl text_size_upr Prompt: Size (m)
      mask DialogControl text_conn_upr Prompt: Connections
      mask DialogControl text_upright Prompt: Upright
      mask DialogControl text_stub_axle Prompt: Stub Axle
      mask DialogControl cont_steer Prompt: Steer
      mask DialogControl grp_rod Prompt: Rod
      mask DialogControl cont_vis_rod Prompt: Visualization
      mask DialogControl text_clr_rod Prompt: Color [RGB]
      mask DialogControl text_opc_rod Prompt: Opac. (0-1)
      mask DialogControl text_size_rod Prompt: Size (m)
      mask DialogControl text_conn_rod Prompt: Connections
      mask DialogControl text_rod_rod Prompt: Rod
      mask DialogControl cont_init Prompt: Initial
  Rack : PMIOPort  Side=Right
  Ref : PMIOPort  Port=2  Side=Right
  Axle : PMIOPort  Port=3  Side=Left
  S : PMIOPort  Port=4  Side=Left
  D : PMIOPort  Port=5  Side=Left
  LAo : PMIOPort  Port=6  Side=Left
  WhlAng : Outport

== system MultibodySuspensionRearSSC/Dampers/Independent/Damper RL/Damper ==
  Ctrl : Inport
  Linear : Subsystem  VariantControl=Linear  mask(Linear Damper with Hard Stop){dam_b=Damper.Damping.d.Value, hp_dpr_top=Damper.Damping.sTop.Value, hp_dpr_bot=Damper.Damping.sBottom.Value, bs_lim_upper=Damper.Endstop.xMax.Value, bs_lim_lower=Damper.Endstop.xMin.Value, bs_k_upper=Damper.Endstop.KxMax.Value, bs_k_lower=Damper.Endstop.KxMin.Value, bs_b_upper=Damper.Endstop.dxMax.Value, bs_b_lower=Damper.Endstop.dxMin.Value, bs_region=Damper.Endstop.xTransition.Value}
      mask prompts: dam_b "Damper (N/(m/s))"; hp_dpr_top "HP Damper Top [xyz] (m)"; hp_dpr_bot "HP Damper Bottom [xyz] (m)"; bs_region "Transition Region (m)"
      mask help: Damper and hard stop with linear behavior with measurements.
      mask init:
      | dam_x0 = norm(hp_dpr_top - hp_dpr_bot);
      mask TypeOptions dam_b: Damper/D
      mask DialogControl text_bumpstop_upper Prompt: Upper
      mask DialogControl text_bumpstop_lower Prompt: Lower
      mask DialogControl text_bumpstop_limit Prompt: Limit (m)
      mask DialogControl text_bumpstop_k Prompt: Stiffness (N/m)
      mask DialogControl text_bumpstop_b Prompt: Damping  (N/(m/s))
  Table : Subsystem  VariantControl=Table  mask(Linear Damper with Hard Stop){dam_bTable=Damper.Damping.dTable.Value, dam_vTable=Damper.Damping.vTable.Value, hp_dpr_top=Damper.Damping.sTop.Value, hp_dpr_bot=Damper.Damping.sBottom.Value, bs_lim_upper=Damper.Endstop.xMax.Value, bs_lim_lower=Damper.Endstop.xMin.Value, bs_k_upper=Damper.Endstop.KxMax.Value, bs_k_lower=Damper.Endstop.KxMin.Value, bs_b_upper=Damper.Endstop.dxMax.Value, bs_b_lower=Damper.Endstop.dxMin.Value, bs_region=Damper.Endstop.xTransition.Value}
      mask prompts: dam_bTable "Damper (N/(m/s))"; dam_vTable "Damper Velocity (m/s)"; hp_dpr_top "HP Damper Top [xyz] (m)"; hp_dpr_bot "HP Damper Bottom [xyz] (m)"; bs_region "Transition Region (m)"
      mask help: Damper and hard stop with linear behavior with measurements.
      mask init:
      | dam_x0 = norm(hp_dpr_top - hp_dpr_bot);
      mask TypeOptions dam_bTable: Damper/D
      mask DialogControl text_bumpstop_upper Prompt: Upper
      mask DialogControl text_bumpstop_lower Prompt: Lower
      mask DialogControl text_bumpstop_limit Prompt: Limit (m)
      mask DialogControl text_bumpstop_k Prompt: Stiffness (N/m)
      mask DialogControl text_bumpstop_b Prompt: Damping  (N/(m/s))
  R : PMIOPort  Side=Left
  C : PMIOPort  Port=2  Side=Right
  meas : Outport

== system MultibodySuspensionRearSSC/Dampers/Independent/Damper RR/Damper ==
  Ctrl : Inport
  Linear : Subsystem  VariantControl=Linear  mask(Linear Damper with Hard Stop){dam_b=Damper.Damping.d.Value, hp_dpr_top=Damper.Damping.sTop.Value, hp_dpr_bot=Damper.Damping.sBottom.Value, bs_lim_upper=Damper.Endstop.xMax.Value, bs_lim_lower=Damper.Endstop.xMin.Value, bs_k_upper=Damper.Endstop.KxMax.Value, bs_k_lower=Damper.Endstop.KxMin.Value, bs_b_upper=Damper.Endstop.dxMax.Value, bs_b_lower=Damper.Endstop.dxMin.Value, bs_region=Damper.Endstop.xTransition.Value}
      mask prompts: dam_b "Damper (N/(m/s))"; hp_dpr_top "HP Damper Top [xyz] (m)"; hp_dpr_bot "HP Damper Bottom [xyz] (m)"; bs_region "Transition Region (m)"
      mask help: Damper and hard stop with linear behavior with measurements.
      mask init:
      | dam_x0 = norm(hp_dpr_top - hp_dpr_bot);
      mask TypeOptions dam_b: Damper/D
      mask DialogControl text_bumpstop_upper Prompt: Upper
      mask DialogControl text_bumpstop_lower Prompt: Lower
      mask DialogControl text_bumpstop_limit Prompt: Limit (m)
      mask DialogControl text_bumpstop_k Prompt: Stiffness (N/m)
      mask DialogControl text_bumpstop_b Prompt: Damping  (N/(m/s))
  Table : Subsystem  VariantControl=Table  mask(Linear Damper with Hard Stop){dam_bTable=Damper.Damping.dTable.Value, dam_vTable=Damper.Damping.vTable.Value, hp_dpr_top=Damper.Damping.sTop.Value, hp_dpr_bot=Damper.Damping.sBottom.Value, bs_lim_upper=Damper.Endstop.xMax.Value, bs_lim_lower=Damper.Endstop.xMin.Value, bs_k_upper=Damper.Endstop.KxMax.Value, bs_k_lower=Damper.Endstop.KxMin.Value, bs_b_upper=Damper.Endstop.dxMax.Value, bs_b_lower=Damper.Endstop.dxMin.Value, bs_region=Damper.Endstop.xTransition.Value}
      mask prompts: dam_bTable "Damper (N/(m/s))"; dam_vTable "Damper Velocity (m/s)"; hp_dpr_top "HP Damper Top [xyz] (m)"; hp_dpr_bot "HP Damper Bottom [xyz] (m)"; bs_region "Transition Region (m)"
      mask help: Damper and hard stop with linear behavior with measurements.
      mask init:
      | dam_x0 = norm(hp_dpr_top - hp_dpr_bot);
      mask TypeOptions dam_bTable: Damper/D
      mask DialogControl text_bumpstop_upper Prompt: Upper
      mask DialogControl text_bumpstop_lower Prompt: Lower
      mask DialogControl text_bumpstop_limit Prompt: Limit (m)
      mask DialogControl text_bumpstop_k Prompt: Stiffness (N/m)
      mask DialogControl text_bumpstop_b Prompt: Damping  (N/(m/s))
  R : PMIOPort  Side=Left
  C : PMIOPort  Port=2  Side=Right
  meas : Outport

== system MultibodySuspensionRearSSC/Springs/Independent/Spring RL/Spring ==
  Ctrl : Inport
  Linear : Subsystem  VariantControl=Linear  mask(Linear Spring){spr_def0=Spring.xPreload.Value, spr_k=Spring.K.Value, spr_hp_top=Spring.sTop.Value, spr_hp_bot=Spring.sBottom.Value}
      mask prompts: spr_def0 "Spr. Preload (m)"; spr_k "Spring Rate (N/m)"; spr_hp_top "HP Top [xyz] (m)"; spr_hp_bot "HP Bottom [xyz] (m)"
      mask help: Spring with linear behavior with measurements.
      mask init:
      | spr_len0 = norm(spr_hp_top-spr_hp_bot);
  Table : Subsystem  VariantControl=Table  mask(Linear Spring){spr_def0=Spring.xPreload.Value, spr_kTable=Spring.KTable.Value, spr_xTable=Spring.xTable.Value, spr_hp_top=Spring.sTop.Value, spr_hp_bot=Spring.sBottom.Value}
      mask prompts: spr_def0 "Spr. Preload (m)"; spr_kTable "Spring Rate (N/m)"; spr_xTable "Spring Deflection (m)"; spr_hp_top "HP Top [xyz] (m)"; spr_hp_bot "HP Bottom [xyz] (m)"
      mask help: Spring with linear behavior with measurements.
      mask init:
      | spr_len0 = norm(spr_hp_top-spr_hp_bot);
  R : PMIOPort  Side=Left
  C : PMIOPort  Port=2  Side=Right
  meas : Outport

== system MultibodySuspensionRearSSC/Springs/Independent/Spring RR/Spring ==
  Ctrl : Inport
  Linear : Subsystem  VariantControl=Linear  mask(Linear Spring){spr_def0=Spring.xPreload.Value, spr_k=Spring.K.Value, spr_hp_top=Spring.sTop.Value, spr_hp_bot=Spring.sBottom.Value}
      mask prompts: spr_def0 "Spr. Preload (m)"; spr_k "Spring Rate (N/m)"; spr_hp_top "HP Top [xyz] (m)"; spr_hp_bot "HP Bottom [xyz] (m)"
      mask help: Spring with linear behavior with measurements.
      mask init:
      | spr_len0 = norm(spr_hp_top-spr_hp_bot);
  Table : Subsystem  VariantControl=Table  mask(Linear Spring){spr_def0=Spring.xPreload.Value, spr_kTable=Spring.KTable.Value, spr_xTable=Spring.xTable.Value, spr_hp_top=Spring.sTop.Value, spr_hp_bot=Spring.sBottom.Value}
      mask prompts: spr_def0 "Spr. Preload (m)"; spr_kTable "Spring Rate (N/m)"; spr_xTable "Spring Deflection (m)"; spr_hp_top "HP Top [xyz] (m)"; spr_hp_bot "HP Bottom [xyz] (m)"
      mask help: Spring with linear behavior with measurements.
      mask init:
      | spr_len0 = norm(spr_hp_top-spr_hp_bot);
  R : PMIOPort  Side=Left
  C : PMIOPort  Port=2  Side=Right
  meas : Outport

== system MultibodySuspensionRearSSC/SuspR/Linkage/Anti Roll Bar/ None ==
  Reference Frame LAoL : sm_lib/Frames and Transforms/Reference Frame
  Reference Frame LAoR : sm_lib/Frames and Transforms/Reference Frame
  Reference Frame Ref : sm_lib/Frames and Transforms/Reference Frame
  LAoL : PMIOPort  Side=Left
  Ref : PMIOPort  Port=2  Side=Left
  LAoR : PMIOPort  Port=3  Side=Left
  connections:
  Reference Frame Ref/RConn1 -- Ref/RConn1
  LAoL/RConn1 -- Reference Frame LAoL/RConn1
  LAoR/RConn1 -- Reference Frame LAoR/RConn1

== system MultibodySuspensionRearSSC/SuspR/Linkage/Anti Roll Bar/Simple ==
  Force Left : sm_lib/Forces and Torques/External Force and Torque  EnableForceX=off  EnableForceY=off  EnableForceZ=on  EnableForce=off  ForceResolutionFrame=AttachedFrame  EnableTorqueX=off  EnableTorqueY=off  EnableTorqueZ=off  EnableTorque=off  TorqueResolutionFrame=AttachedFrame
  Force Right : sm_lib/Forces and Torques/External Force and Torque  EnableForceX=off  EnableForceY=off  EnableForceZ=on  EnableForce=off  ForceResolutionFrame=AttachedFrame  EnableTorqueX=off  EnableTorqueY=off  EnableTorqueZ=off  EnableTorque=off  TorqueResolutionFrame=AttachedFrame
  Gain : Gain  Gain=k
  Gain1 : Gain  Gain=-1
  PS-Simulink Converter : nesl_utility/PS-Simulink Converter  PhysicalDomain=network_engine_domain  SubClassName=ps_output  LeftPortType=input  RightPortType=output  PseudoPeriodic=off  Frequencies=[]  VectorFormat=1-D array  Unit=1  AffineConversion=off
  PS-Simulink Converter1 : nesl_utility/PS-Simulink Converter  PhysicalDomain=network_engine_domain  SubClassName=ps_output  LeftPortType=input  RightPortType=output  PseudoPeriodic=off  Frequencies=[]  VectorFormat=1-D array  Unit=1  AffineConversion=off
  Simulink-PS Converter : nesl_utility/Simulink-PS Converter  PhysicalDomain=network_engine_domain  SubClassName=ps_input  LeftPortType=input  RightPortType=output  PseudoPeriodic=off  Frequencies=[]  NoiseDistribution=none  NoiseParameters=[]  Unit=1  AffineConversion=off  FilteringAndDerivatives=provide  SimscapeFilterOrder=1  InputFilterTimeConstant=0.001  UdotUserProvided=0
  Simulink-PS Converter1 : nesl_utility/Simulink-PS Converter  PhysicalDomain=network_engine_domain  SubClassName=ps_input  LeftPortType=input  RightPortType=output  PseudoPeriodic=off  Frequencies=[]  NoiseDistribution=none  NoiseParameters=[]  Unit=1  AffineConversion=off  FilteringAndDerivatives=provide  SimscapeFilterOrder=1  InputFilterTimeConstant=0.001  UdotUserProvided=0
  Subtract : Sum  Inputs=+-
  Transform Sensor Left : sm_lib/Frames and Transforms/Transform Sensor  MeasurementFrame=Base  RotationSequence=XYX  SenseAngle=off  SenseAxis=off  SenseQ=off  SenseR=off  SenseRotationSequence=off  SenseOmegaX=off  SenseOmegaY=off  SenseOmegaZ=off  SenseOmega=off  SenseQDot=off  SenseRDot=off  SenseRotationSequenceDot=off  SenseAlphaX=off  SenseAlphaY=off  SenseAlphaZ=off  SenseAlpha=off  SenseQDDot=off  SenseRDDot=off  SenseX=off  SenseY=off  SenseZ=on  SenseXYZ=off  SenseRad=off  SenseAzim=off  SenseDist=off  SenseInc=off  SenseXDot=off  SenseYDot=off  SenseZDot=off  SenseXYZDot=off  SenseRadDot=off  SenseAzimDot=off  SenseDistDot=off  SenseIncDot=off  SenseXDDot=off  SenseYDDot=off  SenseZDDot=off  SenseXYZDDot=off  SenseRadDDot=off  SenseAzimDDot=off  SenseDistDDot=off  SenseIncDDot=off
  Transform Sensor Right : sm_lib/Frames and Transforms/Transform Sensor  MeasurementFrame=Base  RotationSequence=XYX  SenseAngle=off  SenseAxis=off  SenseQ=off  SenseR=off  SenseRotationSequence=off  SenseOmegaX=off  SenseOmegaY=off  SenseOmegaZ=off  SenseOmega=off  SenseQDot=off  SenseRDot=off  SenseRotationSequenceDot=off  SenseAlphaX=off  SenseAlphaY=off  SenseAlphaZ=off  SenseAlpha=off  SenseQDDot=off  SenseRDDot=off  SenseX=off  SenseY=off  SenseZ=on  SenseXYZ=off  SenseRad=off  SenseAzim=off  SenseDist=off  SenseInc=off  SenseXDot=off  SenseYDot=off  SenseZDot=off  SenseXYZDot=off  SenseRadDot=off  SenseAzimDot=off  SenseDistDot=off  SenseIncDot=off  SenseXDDot=off  SenseYDDot=off  SenseZDDot=off  SenseXYZDDot=off  SenseRadDDot=off  SenseAzimDDot=off  SenseDistDDot=off  SenseIncDDot=off
  LAoL : PMIOPort  Side=Left
  Ref : PMIOPort  Port=2  Side=Left
  LAoR : PMIOPort  Port=3  Side=Left
  wires:
  PS-Simulink Converter/1 -> Subtract/1
  PS-Simulink Converter1/1 -> Subtract/2
  Subtract/1 -> Gain/1
  Gain/1 -> Simulink-PS Converter/1, Gain1/1
  Gain1/1 -> Simulink-PS Converter1/1
  connections:
  Transform Sensor Right/LConn1 -- Transform Sensor Left/LConn1 -- Ref/RConn1
  Transform Sensor Right/RConn1 -- Force Right/RConn1 -- LAoR/RConn1
  Transform Sensor Left/RConn1 -- Force Left/RConn1 -- LAoL/RConn1
  Transform Sensor Left/RConn2 -- PS-Simulink Converter/LConn1
  Transform Sensor Right/RConn2 -- PS-Simulink Converter1/LConn1
  Simulink-PS Converter/RConn1 -- Force Right/LConn1
  Simulink-PS Converter1/RConn1 -- Force Left/LConn1
